simulink model "Model_test_system_simul"  (R2024b)
settings: Solver=ode45  StartTime=0.0  StopTime=5  RelTol=1e-3
values from neighbouring files (symbols this model uses):
  pulse2deg = 360/2000    (= 0.18)    [Plant_EstimTrialUpdateLAB17_04_25.m]
libraries: simulink x1
settings Model: Creator=Riccardo Grosso  LastModifiedBy=Buton
settings DataIOCC: SaveState=on  ReturnWorkspaceOutputs=off
settings DebuggingCC: AlgebraicLoopMsg=none

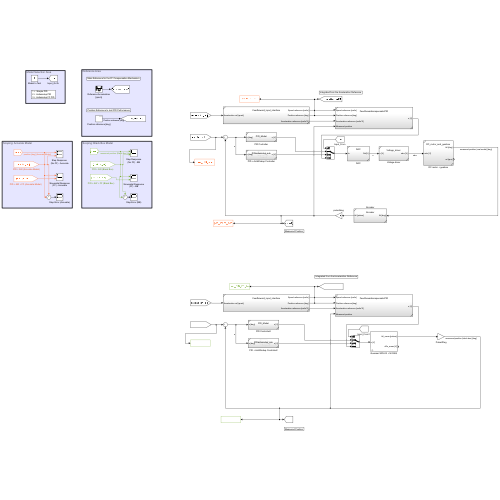
[thumbnail: Simulink's stored preview of the top-level diagram]
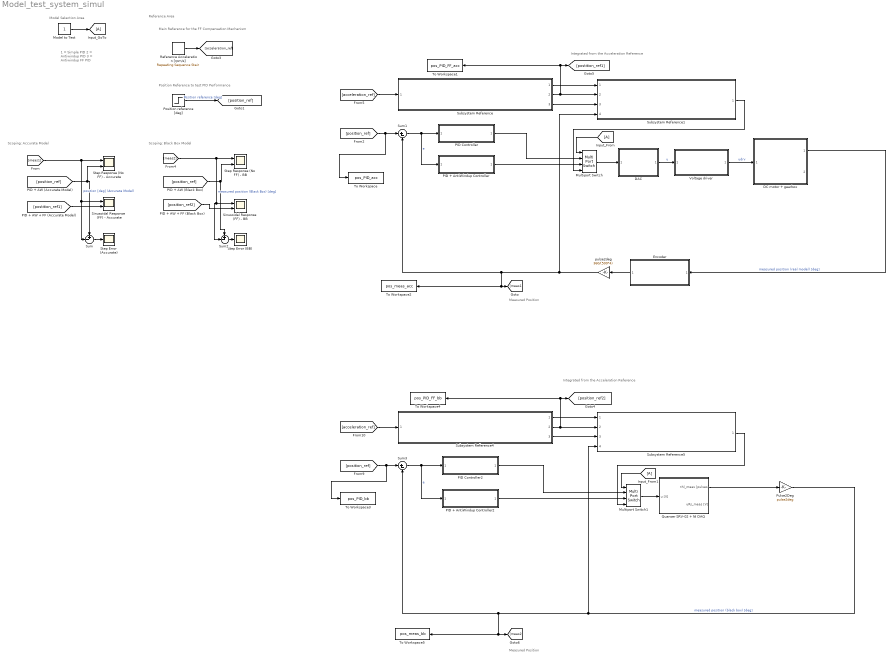
== system Model_test_system_simul ==
  note: Integrated from the Acceleration Reference
  note: Model Selection Area
  note: 1 =  Simple PID
      | 2 =  Antiwindup PID
      | 3 =  Antiwindup FF PID
  note: Reference Area
  note: Main Reference for the FF Compensation Mechanism
  note: Position Reference to test PID Performance
  note: Scoping: Black Box Model
  note: Integrated from the Acceleration Reference
  note: Measured Position
  note: Measured Position
  note: Scoping: Accurate Model
  DAC : Subsystem  ReferencedSubsystem=DAC
  DC motor + gearbox : Subsystem  ReferencedSubsystem=DC_motor_and_gearbox
  Encoder : Subsystem  ReferencedSubsystem=Encoder
  Input_From : From
  Input_From1 : From
  Input_GoTo : Goto
  Model to Test : Constant
  Multiport Switch : MultiPortSwitch  SaturateOnIntegerOverflow=off  InputSameDT=off
  Multiport Switch1 : MultiPortSwitch  SaturateOnIntegerOverflow=off  InputSameDT=off
  PID + AntiWindup Controller : Subsystem  ReferencedSubsystem=PIDantiwindup_sub
  PID + AntiWindup Controller2 : Subsystem  ReferencedSubsystem=PIDantiwindup_sub
  PID Controller : Subsystem  ReferencedSubsystem=PID_Model
  PID Controller2 : Subsystem  ReferencedSubsystem=PID_Model
  Position reference [deg] : Step  Time=0  After=90  SampleTime=0
  Pulse2Deg : Gain  Gain=pulse2deg
  Quanser SRV-02 + NI DAQ : Subsystem  mask(Quanser SRV-02 (with inertial load) + NI DAQ){Ts=0.001, fricType=Karnopp}
      mask prompts: Ts "NI DAQ Sample Time:"; fricType "Friction model"
      mask help: Quanser SRV-02 (with inertial load) + NI DAQ model.
      mask init:
      | %%  Sensors data
      | 
      | %   shunt resistor
      | sens.curr.Rs = 0.5;                         %   resistance [Ohm]   
      | sens.curr.uRs_std = 0.01;                   %   voltage noise standard dev [V]                           
      | sens.curr.uRs_var = sens.curr.uRs_std^2;	%   voltage noise variance [V^2]
      | 
      | %   Hewlett-Packard HEDS-5540#A06 optical encoder
      | sens.enc.ppr = 500*4;                       %   pulses per rotation
      | sens.enc.pulse2deg = 360/sens.enc.ppr;      %   [pulses] -> [deg]
      | sens.enc.pulse2rad = 2*pi/sens.enc.ppr;     %   [pulses] -> [rad]
      | sens.enc.deg2pulse = sens.enc.ppr/360;      %   [deg] -> [pulses]
      | sens.enc.rad2pulse = sens.enc.ppr/2/pi;     %   [rad] -> [pulses]
      | 
      | 
      | %%  Data acquisition board (daq) data
      | 
      | %   NI PCI-6221 DAC data
      | daq.dac.bits = 16;                                  %   resolution (bits)
      | daq.dac.fs   = 10;                                  %   full scale 
      | daq.dac.q    = 2*daq.dac.fs/(2^daq.dac.bits-1);     %	quantization
      | 
      | %   NI PCI-6221 ADC data
      | daq.adc.bits = 16;                                  %   resolution (bits)
      | daq.adc.fs   = 10;                                  %   full scale (as set in SLDRT Analog Input block)
      | daq.adc.q    = 2*daq.adc.fs/(2^daq.adc.bits-1);     %   quantization
      mask Help:
      | Riccardo Antonello (antonello@dei.unipd.it)
      | 
      | April 24, 2020
      | 
      | Dept. of Information Engineering, University of Padova
      mask TypeOptions fricType: Coulomb + viscous | Karnopp
  Reference Acceleration [rpm/s] : simulink/Sources/Repeating Sequence Stair  OutValues=[900 0 -900 -900 0 900].'  tsamp=0.5  OutMin=[]  OutMax=[]  OutDataTypeStr=double  OutputDataTypeScalingMode=double  OutDataType=fixdt(0,8)  ConRadixGroup=Best Precision: Vector-wise  OutScaling=2^-12
  Sinusoidal Response (FF) - Accurate : Scope  NumInputPorts=2
  Sinusoidal Response (FF) - BB : Scope  NumInputPorts=2
  Step Error (Accurate) : Scope
  Step Error (BB) : Scope
  Step Response (No FF) - BB : Scope  NumInputPorts=2
  Step Response (No FF) - Accurate : Scope  NumInputPorts=2
  Subsystem Reference : Subsystem  ReferencedSubsystem=Feedforward_input_interface
  Subsystem Reference1 : Subsystem  ReferencedSubsystem=FeedforwardcompensatorPID
  Subsystem Reference4 : Subsystem  ReferencedSubsystem=Feedforward_input_interface
  Subsystem Reference5 : Subsystem  ReferencedSubsystem=FeedforwardcompensatorPID
  Sum : Sum  Inputs=+-|
  Sum1 : Sum  Inputs=|+-
  Sum2 : Sum  Inputs=+-|
  Sum3 : Sum  Inputs=|+-
  To Workspace : ToWorkspace  VariableName=pos_PID_acc  SaveFormat=Structure With Time  SampleTime=-1
  To Workspace1 : ToWorkspace  VariableName=pos_PID_FF_acc  SaveFormat=Structure With Time  SampleTime=-1
  To Workspace2 : ToWorkspace  VariableName=pos_meas_acc  SaveFormat=Structure With Time  SampleTime=-1
  To Workspace3 : ToWorkspace  VariableName=pos_PID_bb  SaveFormat=Structure With Time  SampleTime=-1
  To Workspace4 : ToWorkspace  VariableName=pos_PID_FF_bb  SaveFormat=Structure With Time  SampleTime=-1
  To Workspace5 : ToWorkspace  VariableName=pos_meas_bb  SaveFormat=Structure With Time  SampleTime=-1
  Voltage driver : Subsystem  ReferencedSubsystem=Voltage_driver
  pulse2deg : Gain  Gain=360/(500*4)
  wires:
  Position reference [deg]/1 -> [position_ref]  "Position reference [deg]"
  DAC/1 -> Voltage driver/1  "u"
  Sum1/1 -> PID + AntiWindup Controller/1, PID Controller/1  "e"
  Encoder/1 -> pulse2deg/1
  DC motor + gearbox/1 -> Encoder/1  "measured position (real model) [deg]"
  Voltage driver/1 -> DC motor + gearbox/1  "udrv"
  Subsystem Reference/3 -> Subsystem Reference1/3
  Subsystem Reference/1 -> Subsystem Reference1/1
  [acceleration_ref] -> Subsystem Reference/1
  Reference Acceleration [rpm/s]/1 -> [acceleration_ref]
  [acceleration_ref] -> Subsystem Reference4/1
  Subsystem Reference4/1 -> Subsystem Reference5/1
  Sum3/1 -> PID + AntiWindup Controller2/1, PID Controller2/1  "e"
  Subsystem Reference4/3 -> Subsystem Reference5/3
  Quanser SRV-02 + NI DAQ/1(thl_meas [pulses]) -> Pulse2Deg/1
  Pulse2Deg/1 -> To Workspace5/1, [meas2], Sum3/2, Subsystem Reference5/4  "measured position (black box) [deg]"
  PID Controller/1 -> Multiport Switch/2
  PID + AntiWindup Controller/1 -> Multiport Switch/3
  Multiport Switch/1 -> DAC/1
  Subsystem Reference1/1 -> Multiport Switch/4
  Input_From/1 -> Multiport Switch/1
  Multiport Switch1/1 -> Quanser SRV-02 + NI DAQ/1(u [V])
  PID + AntiWindup Controller2/1 -> Multiport Switch1/3
  PID Controller2/1 -> Multiport Switch1/2
  Subsystem Reference5/1 -> Multiport Switch1/4
  Input_From1/1 -> Multiport Switch1/1
  Model to Test/1 -> Input_GoTo/1
  pulse2deg/1 -> Subsystem Reference1/4, Sum1/2, To Workspace2/1, [meas1]
  [position_ref] -> To Workspace/1, Sum1/1
  Subsystem Reference/2 -> To Workspace1/1, [postition_ref1], Subsystem Reference1/2
  Subsystem Reference4/2 -> To Workspace4/1, [position_ref2], Subsystem Reference5/2
  [position_ref] -> To Workspace3/1, Sum3/1
  [meas1] -> Sum/2, Sinusoidal Response (FF) - Accurate/1, Step Response (No FF) - Accurate/1  "position [deg] (Accurate Model)"
  [position_ref] -> Sum/1, Step Response (No FF) - Accurate/2
  [postition_ref1] -> Sinusoidal Response (FF) - Accurate/2
  [meas2] -> Sinusoidal Response (FF) - BB/1, Sum2/2, Step Response (No FF) - BB/1  "measured position (Black Box) [deg]"
  [position_ref] -> Sum2/1, Step Response (No FF) - BB/2
  [position_ref2] -> Sinusoidal Response (FF) - BB/2
  Sum/1 -> Step Error (Accurate)/1
  Sum2/1 -> Step Error (BB)/1

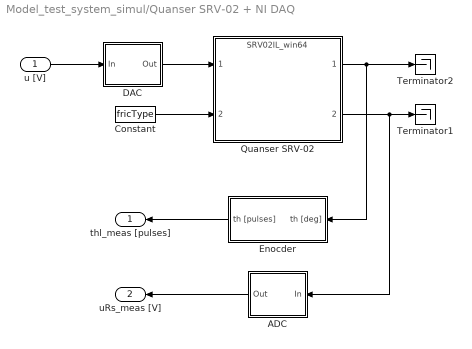
== system Model_test_system_simul/Quanser SRV-02 + NI DAQ ==
  u [V] : Inport
  ADC : Subsystem
  Constant : Constant  Value=fricType
  DAC : Subsystem
  Enocder : Subsystem
  Quanser SRV-02 : ModelReference  ModelNameDialog=SRV02IL_win64.slxp  ModelReferenceVersion=1.44  CopyOfModelProtected=on
  Terminator1 : Terminator
  Terminator2 : Terminator
  thl_meas [pulses] : Outport
  uRs_meas [V] : Outport  Port=2
  wires:
  Enocder/1(th [pulses]) -> thl_meas [pulses]/1
  ADC/1(Out) -> uRs_meas [V]/1
  DAC/1(Out) -> Quanser SRV-02/1
  Quanser SRV-02/2 -> ADC/1(In), Terminator1/1
  u [V]/1 -> DAC/1(In)
  Quanser SRV-02/1 -> Enocder/1(th [deg]), Terminator2/1
  Constant/1 -> Quanser SRV-02/2

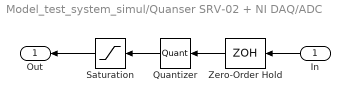
== system Model_test_system_simul/Quanser SRV-02 + NI DAQ/ADC ==
  In : Inport
  Quantizer : Quantizer  QuantizationInterval=daq.adc.q
  Saturation : Saturate  UpperLimit=daq.adc.fs  LowerLimit=-daq.adc.fs
  Zero-Order Hold : ZeroOrderHold  SampleTime=Ts
  Out : Outport
  wires:
  Saturation/1 -> Out/1
  In/1 -> Zero-Order Hold/1
  Quantizer/1 -> Saturation/1
  Zero-Order Hold/1 -> Quantizer/1

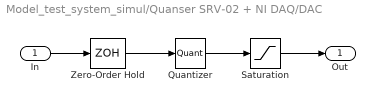
== system Model_test_system_simul/Quanser SRV-02 + NI DAQ/DAC ==
  In : Inport
  Quantizer : Quantizer  QuantizationInterval=daq.dac.q
  Saturation : Saturate  UpperLimit=daq.dac.fs  LowerLimit=-daq.dac.fs
  Zero-Order Hold : ZeroOrderHold  SampleTime=Ts
  Out : Outport
  wires:
  Quantizer/1 -> Saturation/1
  In/1 -> Zero-Order Hold/1
  Zero-Order Hold/1 -> Quantizer/1
  Saturation/1 -> Out/1

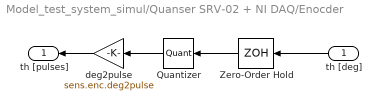
== system Model_test_system_simul/Quanser SRV-02 + NI DAQ/Enocder ==
  th [deg] : Inport
  Quantizer : Quantizer  QuantizationInterval=sens.enc.pulse2deg
  Zero-Order Hold : ZeroOrderHold  SampleTime=Ts
  deg2pulse : Gain  Gain=sens.enc.deg2pulse
  th [pulses] : Outport
  wires:
  Quantizer/1 -> deg2pulse/1
  th [deg]/1 -> Zero-Order Hold/1
  Zero-Order Hold/1 -> Quantizer/1
  deg2pulse/1 -> th [pulses]/1
